simulink model "Assign_Task5and6"  (R2023a)
settings: Solver=ode1  StartTime=0.0  StopTime=30  FixedStep=Ts  MaxStep=Ts  RelTol=1e-3
model workspace (MAT data in the model file):
  wsw = 2000
values from neighbouring files (symbols this model uses):
  fg = 50    [Parameters.m]
  Rtpu = Xtpu/40    (= 0.00375)    [Parameters.m]
  S0non = 1000e6    (= 1000000000)    [Parameters.m]
  Svsc = 100e6    (= 100000000)    [Parameters.m]
  tonvsc = 1e-3    (= 0.001)    [Parameters.m]
  Ts = 20e-6    (= 2e-05)    [Parameters.m]
  Vhv = 22e3    (= 22000)    [Parameters.m]
  Vmv = 22e3    (= 22000)    [Parameters.m]
  wc1 = wsw1/10    (= 848.230016469)    [Parameters.m]
  wpq1 = wc1/10    (= 84.8230016469)    [Parameters.m]
  wsw1 = ksw1*2*pi*fg    (= 8482.30016469)    [Parameters.m]
  Xtpu = 0.15    [Parameters.m]
undefined symbols (not defined in the file or in its folder): D11, Delta, Kf, r, tfilt, theta0
libraries: simulink_extras x20, spsGroundLib x18, spsCurrentMeasurementLib x12, spsVoltageMeasurementLib x12, pid_lib x7, slpidlib x7, spsThreePhaseParallelRLCLoadLib x6, spsControlledVoltageSourceLib x6, powerlib_meascontrol x5, spsThreePhaseBreakerLib x4, eeTransforms x4, spsabctoAlphaBetaZeroLib x3
(part 1 of 3)
settings Model: Creator=Vinicius  LastModifiedBy=citcea
settings SolverCC: AlgebraicLoopSolver=TrustRegion
settings DataIOCC: InitialState=out_EMTsteady50VSC.xFinal  SaveOperatingPoint=on  SaveOutput=off  SignalLogging=off  DSMLogging=off  TimeSaveName=t
settings OptimizationCC: BlockReduction=off
settings ModelReferenceCC: EnableRefExpFcnMdlSchedulingChecks=on
settings RTWCC: BuildConfiguration=Faster Runs  DLArmComputeVersion=19.05

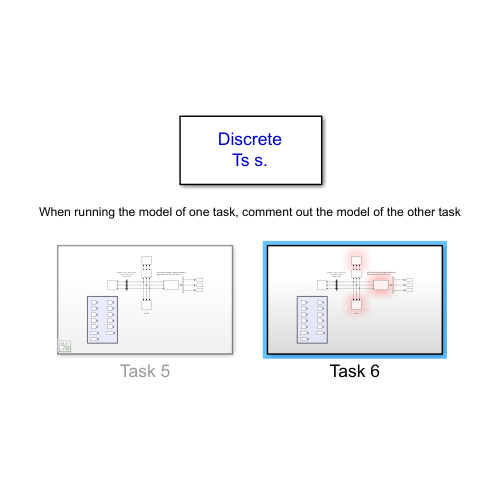
[thumbnail: Simulink's stored preview of the top-level diagram]
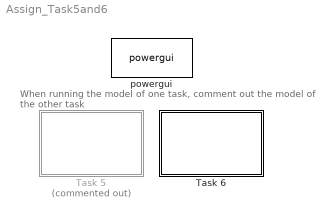
== system Assign_Task5and6 ==
  note: When running the model of one task, comment out the model of the other task
  Task 5 : Subsystem  Commented=on
  Task 6 : Subsystem
  powergui : spspowerguiLib/powergui  Priority=1  SimulationMode=Discrete  SampleTime=Ts  frequency=60  Iterations=50  frequencyindice=50  Pbase=100e6  ErrMax=0.0001  UnitsV=kV  UnitsW=MW  buscounter=0  FunctionMessages=off  echomessages=off  EnableUseOfTLC=off  CurrentSourceSwitches=off  DisableSnubberDevices=off  DisableRonSwitches=off  DisableVfSwitches=off  DisplayEquations=off  AutomaticDiscreteSolvers=off  SolverType=Tustin/Backward Euler (TBE)  Interpol=off  ExternalGateDelay=off  methode=off  Ts=100  x0status=blocks  SPID=on  SwTol=0  HookPort=off  NonlinearTolerance=1e-4  nMaxIteration=100  ContinueOnMaxIteration=off  RestoreLinks=warning  ResistiveCurrentMeasurement=off  Frange=[0:2:500]  Ylog=off  Xlog=on  ShowGrid=off  save=off  variable=ZData  structure=0  ZoomFFT=off  StartTime=0.0  cycles=1  DisplayStyle=1  fundamental=60  FreqAxis=off  MaxFrequency=1000  frequencyindicesteady=1  RmsSteady=1  display=off

== system Assign_Task5and6/Task 5 ==
  note: Variables
  note: Voltage, current, active power and reactive power measurement
  note: Load
  note: active and reactive power setpoints defined inside the VSC block
  Bus : Subsystem
  Bus Selector : BusSelector  OutputSignals=Pabc,Qabc,f
  Generator : Subsystem
      mask Display: disp('SG')
  Load bus 5 : spsThreePhaseParallelRLCLoadLib/Three-Phase Parallel RLC Load  LConnTagsString=A|B|C  Configuration=Y (grounded)  NominalVoltage=Vmv  Vabc=[1e3 1e3 1e3]  Vabcp=[1e3 1e3 1e3]  NominalFrequency=fg  UnbalancedPower=off  ActivePower=300e6  InductivePower=50e6  CapacitivePower=0  Pabc=[10e3 9e3 11e3]  QLabc=[100 90 110]  QCabc=[100 90 110]  Pabcp=[10e3 9e3 11e3]  QLabcp=[100 90 110]  QCabcp=[100 90 110]  Measurements=None  LoadType=constant PQ
  Three-Phase Parallel RLC Load2 : spsThreePhaseParallelRLCLoadLib/Three-Phase Parallel RLC Load  LConnTagsString=A|B|C  Configuration=Y (grounded)  NominalVoltage=Vmv  Vabc=[1 1 1]*Vhv  Vabcp=[1e3 1e3 1e3]  NominalFrequency=fg  UnbalancedPower=off  ActivePower=S0non*0.4  InductivePower=0  CapacitivePower=0  Pabc=[10 10 10]*1e6  QLabc=[1 1 1]*1e6  QCabc=[0 0 0]  Pabcp=[10e3 9e3 11e3]  QLabcp=[100 90 110]  QCabcp=[100 90 110]  Measurements=None  LoadType=constant Z
  Three-Phase Breaker1 : spsThreePhaseBreakerLib/Three-Phase Breaker  InitialState=open  SwitchA=on  SwitchB=on  SwitchC=on  SwitchTimes=4  External=off  BreakerResistance=0.001  SnubberResistance=1e7  SnubberCapacitance=inf  Measurements=None
  VSC : Subsystem  mask{fg=fg, Vhv=Vmv, Vmv=Vmv, Pconv=Svsc, Rtpu=Rtpu, Xtpu=Xtpu, wsw=wsw1, wn_pll=2*pi*80, wc=wc1, wpq=wpq1, koc=1.2}
      mask prompts: fg "AC grid frequency (Hz)"; Vhv "Grid-side voltage (V)(LL-rms)"; Vmv "Converter-side voltage (V)(LL-rms)"; Pconv "Converter nominal power (VA)"; Rtpu "Resistance seen by the converter (p.u)"; Xtpu "Reactance seen by the converter (p.u)"; wsw "Switching frequency (rad/s)"; wn_pll "PLL filter natural frequency"; wc "Current-control bandwidth (rad/s)"; wpq "PQ control bandwidth (rad/s)"; koc "Overcurrent factor (p.u)"
      mask init:
      | %% ----------------------VSC Parameters-------------------------- %%
      | Vmvpk = Vmv*sqrt(2)/sqrt(3);    % Converter-side voltage phase-to-ground peak-to-peak
      | Vhvpk = Vhv*sqrt(2)/sqrt(3);    % Grid-side voltage phase-to-ground peak-to-peak  
      | ksw = round(wsw/(2*pi*fg));      % Calculates switching ratio
      | Iconvbase = 2*Pconv/(3*Vmvpk);  % Converter base current (A)
      | Imax = koc*Iconvbase;   % Converter maximum output current
      | 
      | Xt = Xtpu*(Vmv^2/Pconv);        % p.u to (Ohms)
      | Lt = Xt/(2*pi*fg);              % p.u to (H)
      | Rt = Rtpu*(Vmv^2/Pconv);        % p.u. to (Ohms)
      | 
      | % ------------ PLL ------------- %
      | zeta_pll = 1/sqrt(2);           % Damping
      | kp_pll = 2*zeta_pll*wn_pll/(Vmvpk);
      | tau_pll = 2*zeta_pll/wn_pll;
      | 
      | % ------------ Inner-loop (current control) ------------ %
      | kp_c = Lt*wc; 
      | ti_c = Lt/Rt;
      | 
      | % -------- Outer-loop (voltage and/or power control)
      | % --- PQ closed-loop control ----
      | ti_pq = 1/wc;
      | kp_pq = 2/3*ti_pq*wpq*1/Vmvpk;
      | 
      | 
      | negseq_en = 0;
      mask DialogControl DescTextVar Prompt: Three-phase VSC model
      mask DialogControl Tab1 Prompt: Electrical parameters
      mask DialogControl Tab2 Prompt: Control parameters
      mask Display: disp('VSC')
  tag scope: Pvsc=global, Qvsc=global, fvsc=global
  wires:
  Bus Selector/1 -> [Pvsc]  "<Pabc>"
  Bus Selector/2 -> [Qvsc]  "<Qabc>"
  Bus Selector/3 -> [fvsc]  "<f>"
  VSC/1(m) -> Bus Selector/1
  connections:
  Load bus 5/LConn1 -- Three-Phase Breaker1/LConn1 -- VSC/LConn1 -- Bus/RConn1
  Load bus 5/LConn2 -- Bus/RConn2 -- VSC/LConn2 -- Three-Phase Breaker1/LConn2
  Generator/RConn1 -- Bus/LConn1
  Load bus 5/LConn3 -- Three-Phase Breaker1/LConn3 -- VSC/LConn3 -- Bus/RConn3
  Generator/RConn2 -- Bus/LConn2
  Generator/RConn3 -- Bus/LConn3
  Three-Phase Breaker1/RConn2 -- Three-Phase Parallel RLC Load2/LConn2
  Three-Phase Breaker1/RConn3 -- Three-Phase Parallel RLC Load2/LConn3
  Three-Phase Parallel RLC Load2/LConn1 -- Three-Phase Breaker1/RConn1

== system Assign_Task5and6/Task 6 ==
  note: Variables
  note: Voltage, current, active power and reactive power measurement
  note: Load
  note: active and reactive power setpoints defined inside the VSC block
  Bus : Subsystem
  Bus Selector : BusSelector  OutputSignals=Pabc,Qabc,f
  Generator : Subsystem
      mask Display: disp('SG')
  Load bus 5 : spsThreePhaseParallelRLCLoadLib/Three-Phase Parallel RLC Load  LConnTagsString=A|B|C  Configuration=Y (grounded)  NominalVoltage=Vmv  Vabc=[1e3 1e3 1e3]  Vabcp=[1e3 1e3 1e3]  NominalFrequency=fg  UnbalancedPower=off  ActivePower=300e6  InductivePower=50e6  CapacitivePower=0  Pabc=[10e3 9e3 11e3]  QLabc=[100 90 110]  QCabc=[100 90 110]  Pabcp=[10e3 9e3 11e3]  QLabcp=[100 90 110]  QCabcp=[100 90 110]  Measurements=None  LoadType=constant PQ
  Three-Phase Parallel RLC Load2 : spsThreePhaseParallelRLCLoadLib/Three-Phase Parallel RLC Load  LConnTagsString=A|B|C  Configuration=Y (grounded)  NominalVoltage=Vmv  Vabc=[1 1 1]*Vhv  Vabcp=[1e3 1e3 1e3]  NominalFrequency=fg  UnbalancedPower=off  ActivePower=S0non*0.4  InductivePower=0  CapacitivePower=0  Pabc=[10 10 10]*1e6  QLabc=[1 1 1]*1e6  QCabc=[0 0 0]  Pabcp=[10e3 9e3 11e3]  QLabcp=[100 90 110]  QCabcp=[100 90 110]  Measurements=None  LoadType=constant Z
  Three-Phase Breaker1 : spsThreePhaseBreakerLib/Three-Phase Breaker  InitialState=open  SwitchA=on  SwitchB=on  SwitchC=on  SwitchTimes=4  External=off  BreakerResistance=0.001  SnubberResistance=1e7  SnubberCapacitance=inf  Measurements=None
  VSC : Subsystem  mask{fg=fg, Vhv=Vmv, Vmv=Vmv, Pconv=Svsc, Rtpu=Rtpu, Xtpu=Xtpu, wsw=wsw1, wn_pll=2*pi*80, wc=wc1, wpq=wpq1, koc=1.2}
      mask prompts: fg "AC grid frequency (Hz)"; Vhv "Grid-side voltage (V)(LL-rms)"; Vmv "Converter-side voltage (V)(LL-rms)"; Pconv "Converter nominal power (VA)"; Rtpu "Resistance seen by the converter (p.u)"; Xtpu "Reactance seen by the converter (p.u)"; wsw "Switching frequency (rad/s)"; wn_pll "PLL filter natural frequency"; wc "Current-control bandwidth (rad/s)"; wpq "PQ control bandwidth (rad/s)"; koc "Overcurrent factor (p.u)"
      mask init: same as Assign_Task5and6/Task 5/VSC
      mask DialogControl DescTextVar Prompt: Three-phase VSC model
      mask DialogControl Tab1 Prompt: Electrical parameters
      mask DialogControl Tab2 Prompt: Control parameters
      mask Display: disp('VSC')
  tag scope: Pvsc=global, Qvsc=global, fvsc=global
  wires:
  Bus Selector/1 -> [Pvsc]  "<Pabc>"
  Bus Selector/2 -> [Qvsc]  "<Qabc>"
  Bus Selector/3 -> [fvsc]  "<f>"
  VSC/1(m) -> Bus Selector/1
  connections:
  Three-Phase Breaker1/LConn1 -- Bus/RConn1 -- Load bus 5/LConn1 -- VSC/LConn1
  Bus/RConn2 -- Three-Phase Breaker1/LConn2 -- Load bus 5/LConn2 -- VSC/LConn2
  Generator/RConn1 -- Bus/LConn1
  Three-Phase Breaker1/LConn3 -- Bus/RConn3 -- Load bus 5/LConn3 -- VSC/LConn3
  Generator/RConn2 -- Bus/LConn2
  Generator/RConn3 -- Bus/LConn3
  Three-Phase Breaker1/RConn2 -- Three-Phase Parallel RLC Load2/LConn2
  Three-Phase Breaker1/RConn3 -- Three-Phase Parallel RLC Load2/LConn3
  Three-Phase Parallel RLC Load2/LConn1 -- Three-Phase Breaker1/RConn1

== system Assign_Task5and6/Task 5/Bus ==
  Current Measurement : spsCurrentMeasurementLib/Current Measurement  PhasorSimulation=off  OutputType=Complex  PSBequivalent=0
  Current Measurement1 : spsCurrentMeasurementLib/Current Measurement  PhasorSimulation=off  OutputType=Complex  PSBequivalent=0
  Current Measurement2 : spsCurrentMeasurementLib/Current Measurement  PhasorSimulation=off  OutputType=Complex  PSBequivalent=0
  Ground3 : spsGroundLib/Ground  LConnTagsString=a
  Ground4 : spsGroundLib/Ground  LConnTagsString=a
  Ground5 : spsGroundLib/Ground  LConnTagsString=a
  Mux : Mux  Inputs=3
  Mux1 : Mux  Inputs=3
  Mux2 : Mux  Inputs=2
  "Power (3ph, Instantaneous)" : powerlib_meascontrol/Measurements/Power (3ph, Instantaneous)
  Voltage Measurement : spsVoltageMeasurementLib/Voltage Measurement  PhasorSimulation=off  OutputType=Complex  PSBequivalent=0
  Voltage Measurement2 : spsVoltageMeasurementLib/Voltage Measurement  PhasorSimulation=off  OutputType=Complex  PSBequivalent=0
  Voltage Measurement3 : spsVoltageMeasurementLib/Voltage Measurement  PhasorSimulation=off  OutputType=Complex  PSBequivalent=0
  A : PMIOPort  Side=Left
  B : PMIOPort  Port=2  Side=Left
  C : PMIOPort  Port=3  Side=Left
  a : PMIOPort  Port=4  Side=Right
  b : PMIOPort  Port=5  Side=Right
  c : PMIOPort  Port=6  Side=Right
  tag scope: Ig=global, PQ=global, Vg=global
  wires:
  Voltage Measurement3/1 -> Mux/3
  Voltage Measurement2/1 -> Mux/2
  Voltage Measurement/1 -> Mux/1
  Mux/1 -> [Vg], "Power (3ph, Instantaneous)"/1
  Current Measurement/1 -> Mux1/1
  Current Measurement1/1 -> Mux1/2
  Current Measurement2/1 -> Mux1/3
  Mux1/1 -> [Ig], "Power (3ph, Instantaneous)"/2
  "Power (3ph, Instantaneous)"/1 -> Mux2/1
  "Power (3ph, Instantaneous)"/2 -> Mux2/2
  Mux2/1 -> [PQ]
  connections:
  Ground5/LConn1 -- Voltage Measurement3/LConn2
  Current Measurement/RConn1 -- a/RConn1
  Voltage Measurement2/LConn1 -- Current Measurement1/LConn1 -- B/RConn1
  Voltage Measurement3/LConn1 -- Current Measurement2/LConn1 -- C/RConn1
  Voltage Measurement/LConn1 -- Current Measurement/LConn1 -- A/RConn1
  Ground3/LConn1 -- Voltage Measurement/LConn2
  Ground4/LConn1 -- Voltage Measurement2/LConn2
  Current Measurement1/RConn1 -- b/RConn1
  Current Measurement2/RConn1 -- c/RConn1

== system Assign_Task5and6/Task 5/Generator ==
  note: The Snubber should be at least equal to 1% of the machine power to avoid numerical oscillations
  note: Nomenclature:
      |
      | Pm = mechanical power provided to the generator
      | Tm = mechanical torque provided to the generator
      | wm = mechanical speed in p.u
      | dw = speed variation (wm-1) in p.u
      | Efd = Exciter output voltage (generator field voltage)
      | Ifd = Exciter output current (generator field current)
      | Vt = Generator terminal voltage
      | It = Generator terminal current
      | Vref = Voltage regulator reference signal
  note: Synchronous Machine Model according to ENTSO-E
  note: The mechanical power should be changed here in this constant and also in the turbine parameters
  Abs1 : Abs  SaturateOnIntegerOverflow=off
  Abs2 : Abs  SaturateOnIntegerOverflow=off
  Bus Selector : BusSelector  OutputSignals=dw,w,vq,vd,iq,id,Peo,Te,ifd
  Divide : Product  Inputs=*/
  Exciter : Subsystem  mask{K=200, Ta=3, Tb=10, Te=0.05, Emin=-4, Emax=4, Vf0=1.30534}
      mask prompts: K "Controller gain (K)"; Ta "Filter derivative time constant (Ta)(sec)"; Tb "Filter delay time (Tb)(sec)"; Te "Exciter time constant (Te)(sec)"; Emin "Controller minimum output (Emin)"; Emax "Controller maximum output (Emax)"; Vf0 "Initial output (p.u)"
      mask Display:
      | disp('AVR')
      | 
      | port_label('input',1,'Vref')
      | port_label('input',2,'Vc')
      | 
      | port_label('output',1,'Efd')
  Mech power (p.u) : Constant  Value=0.350  VectorParams1D=off
  Real-Imag to Complex : RealImagToComplex
  Real-Imag to Complex1 : RealImagToComplex
  Scope : Scope
  Snubber : spsThreePhaseParallelRLCLoadLib/Three-Phase Parallel RLC Load  LConnTagsString=A|B|C  Configuration=Y (grounded)  NominalVoltage=Vmv  Vabc=[1 1 1]*Vmv  Vabcp=[1e3 1e3 1e3]  NominalFrequency=fg  UnbalancedPower=off  ActivePower=0.05*S0non  InductivePower=0  CapacitivePower=0  Pabc=[10e3 10e3 10e3]  QLabc=[0 0 0]  QCabc=[0 0 0]  Pabcp=[10e3 9e3 11e3]  QLabcp=[100 90 110]  QCabcp=[100 90 110]  Measurements=None  LoadType=constant Z
  Synchronous machine : spsSynchronousMachinepuStandardLib/Synchronous Machine pu Standard  PresetModel=No  MechanicalLoad=Mechanical power Pm  ShowDetailedParameters=on  RotorType=Salient-pole  Units=per unit standard parameters  MeasurementBus=on  NominalParameters=[S0non Vmv fg]  Reactances1=[ 1.81, 0.3, 0.23, 1.76, 0.65, 0.25, 0.15 ]  Reactances2=[2.0 0.35 0.25 1.8 0.3 0.15]  dAxisTimeConstants=Short-circuit  qAxisTimeConstants=Short-circuit  TimeConstants1="[ 4.4849  0.0681  0.1  ]"  TimeConstants2=[ 8.0, 0.03, 1.0, 0.07 ]  TimeConstants3="[  4.49  0.0681  0.0513  ]"  TimeConstants4=[ 8.0, 0.03, 0.3371, 0.0295 ]  TimeConstants5=[ 1.01, 0.053, 0.1 ]  TimeConstants6=[ 1.3201, 0.023, 1.0, 0.07 ]  TimeConstants7=[0.9 0.03 0.05]  TimeConstants8=[ 1.3201, 0.0231, 0.3371, 0.0295 ]  StatorResistance=0.01  Mechanical=[6 0 2]  PolePairs=20  InitialConditions=[0 -60.0721 0.353553 0.353553 0.353553 -8.1301 -128.13 111.87 1.30534]  SetSaturation=off  Saturation=[0.6404,0.7127,0.8441,0.9214,0.9956,1.082,1.19,1.316,1.457;0.7,0.7698,0.8872,0.9466,0.9969,1.046,1.1,1.151,1.201]  LoadFlowParameters=[2 47500000 0 0 0]  TsPowergui=0  TsBlock=-1  IterativeModel=Trapezoidal non iterative  IterativeDiscreteModel=Trapezoidal non iterative  BusType=swing  Pref=475e6  Qref=0  Qmin=-inf  Qmax=inf  PLF=0  QLF=0
  Turbine without governor : Subsystem  mask{R=0.05, T1=0.5, T2=3, T3=10, Dt=0, Vmin=0, Vmax=10, P0=0.351}
      mask prompts: R "Controller droop (R)"; T1 "Governor time constant (T1)(sec)"; T2 "Turbine derivative time constant (T2)(sec)"; T3 "Turbine delay time constant (T3)(sec)"; Dt "Frictional losses factor (Dt)"; Vmin "Minimum gate limit (Vmin)(p.u)"; Vmax "Maximum gate limit (Vmax)(p.u)"; P0 "Initial power (p.u)"
      mask Display:
      | disp('Turbine')
      | 
      | port_label('input',1,'Pref')
      | 
      | port_label('output',1,'Pm')
  Voltage ref (p.u) : Constant  Value=1.0
  A : PMIOPort  Side=Right
  B : PMIOPort  Port=2  Side=Right
  C : PMIOPort  Port=3  Side=Right
  tag scope: Efd=global, Ifd=global, It=global, Pe=global, Pm=global, Te=global, Tm=global, Vt=global, dw=global, wm=global
  wires:
  Exciter/1(Efd) -> Synchronous machine/2, [Efd]
  Voltage ref (p.u)/1 -> Exciter/1(Vref)
  Turbine without governor/1(Pm) -> Synchronous machine/1, [Pm]
  Mech power (p.u)/1 -> Turbine without governor/1(RefL)
  [Pm] -> Divide/1
  [wm] -> Divide/2
  Divide/1 -> [Tm]
  Bus Selector/4 -> Real-Imag to Complex/2  "<vd>"
  Abs2/1 -> [It]
  Real-Imag to Complex1/1 -> Abs2/1
  Real-Imag to Complex/1 -> Abs1/1
  Bus Selector/6 -> Real-Imag to Complex1/2  "<id>"
  Bus Selector/2 -> Scope/1, [wm]  "<w>"
  Bus Selector/8 -> [Te]  "<Te>"
  Bus Selector/3 -> Real-Imag to Complex/1  "<vq>"
  Bus Selector/7 -> [Pe]  "<Peo>"
  Bus Selector/5 -> Real-Imag to Complex1/1  "<iq>"
  Synchronous machine/1 -> Bus Selector/1
  Bus Selector/9 -> [Ifd]  "<ifd>"
  Abs1/1 -> [Vt]
  [Vt] -> Exciter/2(Vt)
  Bus Selector/1 -> [dw]  "<dw>"
  connections:
  B/RConn1 -- Synchronous machine/RConn2 -- Snubber/LConn2
  C/RConn1 -- Synchronous machine/RConn3 -- Snubber/LConn3
  Snubber/LConn1 -- Synchronous machine/RConn1 -- A/RConn1

== system Assign_Task5and6/Task 5/VSC ==
  note: Load convention used:
      | positive power = converter absorbs power from the grid
      | negative power = converter injects power into the grid
  Block : Step  Time=4*tonvsc  Before=1  After=0  SampleTime=0
  Electrical part : Subsystem  VariantControl=EMT_AVG
      settings: PortSchema="{\"entries\":[{\"content\":{\"sides\":[{\"content\":{\"connectorIds\":[\"LConn1\",\"LConn2\",\"LConn3\"]},\"type\":\"ConnectorPlacement.EquallySpacedRectSide\",\"uuid\":\"96043b84-a665-4cb2-a938-d6633d7ee474\"},{\"content\":{\"connectorIds\":[\"In1\"],\"side\":\"RIGHT\"},\"type\":\"ConnectorPlacement.EquallySpacedRectSide\",\"uuid\":\"064d463f-c23a-42ac-89ce-8dea3d446214\"},{\"content\":{\"connectorIds\":[],\"side\":\"TOP\"},\"type\":\"ConnectorPlacement.EquallySpacedRectSide\",\"uuid\":\"95ef669c-c6ed-44c3-8b69-447906728b6d\"}]},\"type\":\"ConnectorPlacement.EquallySpacedConnector\",\"uuid\":\"ea66db09-64d7-4d7e-ba7b-d769c56e2dbd\"}],\"packageUris\":[\"http://schema.mathworks.com/mf0/Connector/19700101\"],\"version\":\"1.0\"}"
  NOT : Logic  Operator=NOT  IconShape=distinctive  AllPortsSameDT=off  OutDataTypeStr=boolean
  Pset : Step  Time=4*tonvsc  After=-Svsc*0.2  SampleTime=0
  Qset : Step  Time=tonvsc  After=0  SampleTime=0
  Three-Phase Breaker : spsThreePhaseBreakerLib/Three-Phase Breaker  InitialState=open  SwitchA=on  SwitchB=on  SwitchC=on  SwitchTimes="[1/60  5/60]"  External=on  BreakerResistance=0.001  SnubberResistance=1e7  SnubberCapacitance=inf  Measurements=None
  VI measurement : Subsystem
      settings: PortSchema="{\"entries\":[{\"content\":{\"sides\":[{\"content\":{\"connectorIds\":[\"LConn1\",\"LConn2\",\"LConn3\"]},\"type\":\"ConnectorPlacement.EquallySpacedRectSide\",\"uuid\":\"d0d5b0b8-afec-4f90-9eba-536a06b10059\"},{\"content\":{\"connectorIds\":[\"RConn1\",\"RConn2\",\"RConn3\"],\"side\":\"RIGHT\"},\"type\":\"ConnectorPlacement.EquallySpacedRectSide\",\"uuid\":\"adc1b68d-6172-4507-b54b-9373921355a1\"},{\"content\":{\"connectorIds\":[\"Out1\",\"Out2\"],\"side\":\"TOP\"},\"type\":\"ConnectorPlacement.EquallySpacedRectSide\",\"uuid\":\"8c5adf07-e95b-4907-94c3-1b2a47d47f40\"}]},\"type\":\"ConnectorPlacement.EquallySpacedConnector\",\"uuid\":\"87d0b20f-8f85-4790-a611-3415e642a83a\"}],\"packageUris\":[\"http://schema.mathworks.com/mf0/Connector/R2020b\"],\"version\":\"1.0\"}"
  VSC Control : Subsystem
      settings: PortSchema="{\"entries\":[{\"content\":{\"sides\":[{\"content\":{\"connectorIds\":[\"In1\",\"In2\",\"In3\",\"In4\",\"In5\"]},\"type\":\"ConnectorPlacement.EquallySpacedRectSide\",\"uuid\":\"cada8d9e-53e0-4197-9386-6c7b6ea13844\"},{\"content\":{\"connectorIds\":[\"Out1\"],\"side\":\"RIGHT\"},\"type\":\"ConnectorPlacement.EquallySpacedRectSide\",\"uuid\":\"f237b52a-0d77-45c0-937d-32cafba1283e\"},{\"content\":{\"connectorIds\":[\"Out2\"],\"side\":\"TOP\"},\"type\":\"ConnectorPlacement.EquallySpacedRectSide\",\"uuid\":\"e6f268b5-5f09-49a6-9529-b1aeebd5f021\"}]},\"type\":\"ConnectorPlacement.EquallySpacedConnector\",\"uuid\":\"4d1d2957-2eb9-4111-8c87-957e800b2b0b\"}],\"packageUris\":[\"http://schema.mathworks.com/mf0/Connector/19700101\"],\"version\":\"1.0\"}"
  output signals : Subsystem
  A : PMIOPort  Side=Left
  B : PMIOPort  Port=2  Side=Left
  C : PMIOPort  Port=3  Side=Left
  m : Outport
  wires:
  NOT/1 -> Three-Phase Breaker/1
  VSC Control/1(Ref) -> Electrical part/1(Ref)
  [Is] -> VSC Control/3(Iabc)
  [Vs] -> VSC Control/2(Vabc)
  Block/1 -> VSC Control/1(Block), NOT/1
  [Vs] -> output signals/1(Vs)
  [Is] -> output signals/2(Is)
  VSC Control/2(m) -> output signals/3(control)
  output signals/1(m) -> m/1
  VI measurement/1(Vs) -> [Vs]
  VI measurement/2(Is) -> [Is]
  Pset/1 -> VSC Control/4(Pset)
  Qset/1 -> VSC Control/5(Qset)
  connections:
  Electrical part/LConn3 -- Three-Phase Breaker/LConn3
  Electrical part/LConn2 -- Three-Phase Breaker/LConn2
  Electrical part/LConn1 -- Three-Phase Breaker/LConn1
  Three-Phase Breaker/RConn1 -- VI measurement/RConn1
  Three-Phase Breaker/RConn2 -- VI measurement/RConn2
  Three-Phase Breaker/RConn3 -- VI measurement/RConn3
  VI measurement/LConn3 -- C/RConn1
  A/RConn1 -- VI measurement/LConn1
  B/RConn1 -- VI measurement/LConn2

== system Assign_Task5and6/Task 6/Bus ==
  Current Measurement : spsCurrentMeasurementLib/Current Measurement  PhasorSimulation=off  OutputType=Complex  PSBequivalent=0
  Current Measurement1 : spsCurrentMeasurementLib/Current Measurement  PhasorSimulation=off  OutputType=Complex  PSBequivalent=0
  Current Measurement2 : spsCurrentMeasurementLib/Current Measurement  PhasorSimulation=off  OutputType=Complex  PSBequivalent=0
  Ground3 : spsGroundLib/Ground  LConnTagsString=a
  Ground4 : spsGroundLib/Ground  LConnTagsString=a
  Ground5 : spsGroundLib/Ground  LConnTagsString=a
  Mux : Mux  Inputs=3
  Mux1 : Mux  Inputs=3
  Mux2 : Mux  Inputs=2
  "Power (3ph, Instantaneous)" : spsPower3phInstantaneousLib/Power (3ph, Instantaneous)
  Voltage Measurement : spsVoltageMeasurementLib/Voltage Measurement  PhasorSimulation=off  OutputType=Complex  PSBequivalent=0
  Voltage Measurement2 : spsVoltageMeasurementLib/Voltage Measurement  PhasorSimulation=off  OutputType=Complex  PSBequivalent=0
  Voltage Measurement3 : spsVoltageMeasurementLib/Voltage Measurement  PhasorSimulation=off  OutputType=Complex  PSBequivalent=0
  A : PMIOPort  Side=Left
  B : PMIOPort  Port=2  Side=Left
  C : PMIOPort  Port=3  Side=Left
  a : PMIOPort  Port=4  Side=Right
  b : PMIOPort  Port=5  Side=Right
  c : PMIOPort  Port=6  Side=Right
  tag scope: Ig=global, PQ=global, Vg=global
  wires:
  Voltage Measurement3/1 -> Mux/3
  Voltage Measurement2/1 -> Mux/2
  Voltage Measurement/1 -> Mux/1
  Mux/1 -> [Vg], "Power (3ph, Instantaneous)"/1
  Current Measurement/1 -> Mux1/1
  Current Measurement1/1 -> Mux1/2
  Current Measurement2/1 -> Mux1/3
  Mux1/1 -> [Ig], "Power (3ph, Instantaneous)"/2
  "Power (3ph, Instantaneous)"/1 -> Mux2/1
  "Power (3ph, Instantaneous)"/2 -> Mux2/2
  Mux2/1 -> [PQ]
  connections:
  Ground5/LConn1 -- Voltage Measurement3/LConn2
  Current Measurement/RConn1 -- a/RConn1
  Voltage Measurement2/LConn1 -- Current Measurement1/LConn1 -- B/RConn1
  Voltage Measurement3/LConn1 -- Current Measurement2/LConn1 -- C/RConn1
  Voltage Measurement/LConn1 -- Current Measurement/LConn1 -- A/RConn1
  Ground3/LConn1 -- Voltage Measurement/LConn2
  Ground4/LConn1 -- Voltage Measurement2/LConn2
  Current Measurement1/RConn1 -- b/RConn1
  Current Measurement2/RConn1 -- c/RConn1

== system Assign_Task5and6/Task 6/Generator ==
  note: The Snubber should be at least equal to 1% of the machine power to avoid numerical oscillations
  note: Nomenclature:
      |
      | Pm = mechanical power provided to the generator
      | Tm = mechanical torque provided to the generator
      | wm = mechanical speed in p.u
      | dw = speed variation (wm-1) in p.u
      | Efd = Exciter output voltage (generator field voltage)
      | Ifd = Exciter output current (generator field current)
      | Vt = Generator terminal voltage
      | It = Generator terminal current
      | Vref = Voltage regulator reference signal
  note: Synchronous Machine Model according to ENTSO-E
  note: The mechanical power should be changed here in this constant and also in the turbine parameters
  Abs1 : Abs  SaturateOnIntegerOverflow=off
  Abs2 : Abs  SaturateOnIntegerOverflow=off
  Bus Selector : BusSelector  OutputSignals=dw,w,vq,vd,iq,id,Peo,Te,ifd
  Divide : Product  Inputs=*/
  Exciter : Subsystem  mask{K=200, Ta=3, Tb=10, Te=0.05, Emin=-4, Emax=4, Vf0=1.30534}
      mask prompts: K "Controller gain (K)"; Ta "Filter derivative time constant (Ta)(sec)"; Tb "Filter delay time (Tb)(sec)"; Te "Exciter time constant (Te)(sec)"; Emin "Controller minimum output (Emin)"; Emax "Controller maximum output (Emax)"; Vf0 "Initial output (p.u)"
      mask Display:
      | disp('AVR')
      | 
      | port_label('input',1,'Vref')
      | port_label('input',2,'Vc')
      | 
      | port_label('output',1,'Efd')
  Mech power (p.u) : Constant  Value=0.350  VectorParams1D=off
  Real-Imag to Complex : RealImagToComplex
  Real-Imag to Complex1 : RealImagToComplex
  Scope : Scope
  Snubber : spsThreePhaseParallelRLCLoadLib/Three-Phase Parallel RLC Load  LConnTagsString=A|B|C  Configuration=Y (grounded)  NominalVoltage=Vmv  Vabc=[1 1 1]*Vmv  Vabcp=[1e3 1e3 1e3]  NominalFrequency=fg  UnbalancedPower=off  ActivePower=0.05*S0non  InductivePower=0  CapacitivePower=0  Pabc=[10e3 10e3 10e3]  QLabc=[0 0 0]  QCabc=[0 0 0]  Pabcp=[10e3 9e3 11e3]  QLabcp=[100 90 110]  QCabcp=[100 90 110]  Measurements=None  LoadType=constant Z
  Synchronous machine : spsSynchronousMachinepuStandardLib/Synchronous Machine pu Standard  PresetModel=No  MechanicalLoad=Mechanical power Pm  ShowDetailedParameters=on  RotorType=Salient-pole  Units=per unit standard parameters  MeasurementBus=on  NominalParameters=[S0non Vmv fg]  Reactances1=[ 1.81, 0.3, 0.23, 1.76, 0.65, 0.25, 0.15 ]  Reactances2=[2.0 0.35 0.25 1.8 0.3 0.15]  dAxisTimeConstants=Short-circuit  qAxisTimeConstants=Short-circuit  TimeConstants1="[ 4.4849  0.0681  0.1  ]"  TimeConstants2=[ 8.0, 0.03, 1.0, 0.07 ]  TimeConstants3="[  4.49  0.0681  0.0513  ]"  TimeConstants4=[ 8.0, 0.03, 0.3371, 0.0295 ]  TimeConstants5=[ 1.01, 0.053, 0.1 ]  TimeConstants6=[ 1.3201, 0.023, 1.0, 0.07 ]  TimeConstants7=[0.9 0.03 0.05]  TimeConstants8=[ 1.3201, 0.0231, 0.3371, 0.0295 ]  StatorResistance=0.01  Mechanical=[6 0 2]  PolePairs=20  InitialConditions=[0 -60.0721 0.353553 0.353553 0.353553 -8.1301 -128.13 111.87 1.30534]  SetSaturation=off  Saturation=[0.6404,0.7127,0.8441,0.9214,0.9956,1.082,1.19,1.316,1.457;0.7,0.7698,0.8872,0.9466,0.9969,1.046,1.1,1.151,1.201]  LoadFlowParameters=[2 47500000 0 0 0]  TsPowergui=0  TsBlock=-1  IterativeModel=Trapezoidal non iterative  IterativeDiscreteModel=Trapezoidal non iterative  BusType=swing  Pref=475e6  Qref=0  Qmin=-inf  Qmax=inf  PLF=0  QLF=0
  Turbine without governor : Subsystem  mask{R=0.05, T1=0.5, T2=3, T3=10, Dt=0, Vmin=0, Vmax=10, P0=0.351}
      mask prompts: R "Controller droop (R)"; T1 "Governor time constant (T1)(sec)"; T2 "Turbine derivative time constant (T2)(sec)"; T3 "Turbine delay time constant (T3)(sec)"; Dt "Frictional losses factor (Dt)"; Vmin "Minimum gate limit (Vmin)(p.u)"; Vmax "Maximum gate limit (Vmax)(p.u)"; P0 "Initial power (p.u)"
      mask Display:
      | disp('Turbine')
      | 
      | port_label('input',1,'Pref')
      | 
      | port_label('output',1,'Pm')
  Voltage ref (p.u) : Constant  Value=1.0
  A : PMIOPort  Side=Right
  B : PMIOPort  Port=2  Side=Right
  C : PMIOPort  Port=3  Side=Right
  tag scope: Efd=global, Ifd=global, It=global, Pe=global, Pm=global, Te=global, Tm=global, Vt=global, dw=global, wm=global
  wires:
  Exciter/1(Efd) -> Synchronous machine/2, [Efd]
  Voltage ref (p.u)/1 -> Exciter/1(Vref)
  Turbine without governor/1(Pm) -> Synchronous machine/1, [Pm]
  Mech power (p.u)/1 -> Turbine without governor/1(RefL)
  [Pm] -> Divide/1
  [wm] -> Divide/2
  Divide/1 -> [Tm]
  Bus Selector/4 -> Real-Imag to Complex/2  "<vd>"
  Abs2/1 -> [It]
  Real-Imag to Complex1/1 -> Abs2/1
  Real-Imag to Complex/1 -> Abs1/1
  Bus Selector/6 -> Real-Imag to Complex1/2  "<id>"
  Bus Selector/2 -> Scope/1, [wm]  "<w>"
  Bus Selector/8 -> [Te]  "<Te>"
  Bus Selector/3 -> Real-Imag to Complex/1  "<vq>"
  Bus Selector/7 -> [Pe]  "<Peo>"
  Bus Selector/5 -> Real-Imag to Complex1/1  "<iq>"
  Synchronous machine/1 -> Bus Selector/1
  Bus Selector/9 -> [Ifd]  "<ifd>"
  Abs1/1 -> [Vt]
  [Vt] -> Exciter/2(Vt)
  Bus Selector/1 -> [dw]  "<dw>"
  connections:
  B/RConn1 -- Synchronous machine/RConn2 -- Snubber/LConn2
  C/RConn1 -- Synchronous machine/RConn3 -- Snubber/LConn3
  Snubber/LConn1 -- Synchronous machine/RConn1 -- A/RConn1

== system Assign_Task5and6/Task 6/VSC ==
  note: droop signal goes here
  note: Load convention used:
      | positive power = converter absorbs power from the grid
      | negative power = converter injects power into the grid
  Block : Step  Time=4*tonvsc  Before=1  After=0  SampleTime=0
  Electrical part : Subsystem  VariantControl=EMT_AVG
      settings: PortSchema="{\"entries\":[{\"content\":{\"sides\":[{\"content\":{\"connectorIds\":[\"LConn1\",\"LConn2\",\"LConn3\"]},\"type\":\"ConnectorPlacement.EquallySpacedRectSide\",\"uuid\":\"96043b84-a665-4cb2-a938-d6633d7ee474\"},{\"content\":{\"connectorIds\":[\"In1\"],\"side\":\"RIGHT\"},\"type\":\"ConnectorPlacement.EquallySpacedRectSide\",\"uuid\":\"064d463f-c23a-42ac-89ce-8dea3d446214\"},{\"content\":{\"connectorIds\":[],\"side\":\"TOP\"},\"type\":\"ConnectorPlacement.EquallySpacedRectSide\",\"uuid\":\"95ef669c-c6ed-44c3-8b69-447906728b6d\"}]},\"type\":\"ConnectorPlacement.EquallySpacedConnector\",\"uuid\":\"ea66db09-64d7-4d7e-ba7b-d769c56e2dbd\"}],\"packageUris\":[\"http://schema.mathworks.com/mf0/Connector/19700101\"],\"version\":\"1.0\"}"
  NOT : Logic  Operator=NOT  IconShape=distinctive  AllPortsSameDT=off  OutDataTypeStr=boolean
  Pset : Step  Time=4*tonvsc  After=-Svsc*0.2  SampleTime=0
  Qset : Step  Time=tonvsc  After=0  SampleTime=0
  Three-Phase Breaker : spsThreePhaseBreakerLib/Three-Phase Breaker  InitialState=open  SwitchA=on  SwitchB=on  SwitchC=on  SwitchTimes="[1/60  5/60]"  External=on  BreakerResistance=0.001  SnubberResistance=1e7  SnubberCapacitance=inf  Measurements=None
  VI measurement : Subsystem
      settings: PortSchema="{\"entries\":[{\"content\":{\"sides\":[{\"content\":{\"connectorIds\":[\"LConn1\",\"LConn2\",\"LConn3\"]},\"type\":\"ConnectorPlacement.EquallySpacedRectSide\",\"uuid\":\"d0d5b0b8-afec-4f90-9eba-536a06b10059\"},{\"content\":{\"connectorIds\":[\"RConn1\",\"RConn2\",\"RConn3\"],\"side\":\"RIGHT\"},\"type\":\"ConnectorPlacement.EquallySpacedRectSide\",\"uuid\":\"adc1b68d-6172-4507-b54b-9373921355a1\"},{\"content\":{\"connectorIds\":[\"Out1\",\"Out2\"],\"side\":\"TOP\"},\"type\":\"ConnectorPlacement.EquallySpacedRectSide\",\"uuid\":\"8c5adf07-e95b-4907-94c3-1b2a47d47f40\"}]},\"type\":\"ConnectorPlacement.EquallySpacedConnector\",\"uuid\":\"87d0b20f-8f85-4790-a611-3415e642a83a\"}],\"packageUris\":[\"http://schema.mathworks.com/mf0/Connector/R2020b\"],\"version\":\"1.0\"}"
  VSC Control : Subsystem
      settings: PortSchema="{\"entries\":[{\"content\":{\"sides\":[{\"content\":{\"connectorIds\":[\"In1\",\"In2\",\"In3\",\"In4\",\"In5\"]},\"type\":\"ConnectorPlacement.EquallySpacedRectSide\",\"uuid\":\"cada8d9e-53e0-4197-9386-6c7b6ea13844\"},{\"content\":{\"connectorIds\":[\"Out1\"],\"side\":\"RIGHT\"},\"type\":\"ConnectorPlacement.EquallySpacedRectSide\",\"uuid\":\"f237b52a-0d77-45c0-937d-32cafba1283e\"},{\"content\":{\"connectorIds\":[\"Out2\"],\"side\":\"TOP\"},\"type\":\"ConnectorPlacement.EquallySpacedRectSide\",\"uuid\":\"e6f268b5-5f09-49a6-9529-b1aeebd5f021\"}]},\"type\":\"ConnectorPlacement.EquallySpacedConnector\",\"uuid\":\"4d1d2957-2eb9-4111-8c87-957e800b2b0b\"}],\"packageUris\":[\"http://schema.mathworks.com/mf0/Connector/19700101\"],\"version\":\"1.0\"}"
  output signals : Subsystem
  A : PMIOPort  Side=Left
  B : PMIOPort  Port=2  Side=Left
  C : PMIOPort  Port=3  Side=Left
  m : Outport
  wires:
  NOT/1 -> Three-Phase Breaker/1
  VSC Control/1(Ref) -> Electrical part/1(Ref)
  [Is] -> VSC Control/3(Iabc)
  [Vs] -> VSC Control/2(Vabc)
  Block/1 -> VSC Control/1(Block), NOT/1
  [Vs] -> output signals/1(Vs)
  [Is] -> output signals/2(Is)
  VSC Control/2(m) -> output signals/3(control)
  output signals/1(m) -> m/1
  VI measurement/1(Vs) -> [Vs]
  VI measurement/2(Is) -> [Is]
  Pset/1 -> VSC Control/4(Pset)
  Qset/1 -> VSC Control/5(Qset)
  connections:
  Electrical part/LConn3 -- Three-Phase Breaker/LConn3
  Electrical part/LConn2 -- Three-Phase Breaker/LConn2
  Electrical part/LConn1 -- Three-Phase Breaker/LConn1
  Three-Phase Breaker/RConn1 -- VI measurement/RConn1
  Three-Phase Breaker/RConn2 -- VI measurement/RConn2
  Three-Phase Breaker/RConn3 -- VI measurement/RConn3
  VI measurement/LConn3 -- C/RConn1
  A/RConn1 -- VI measurement/LConn1
  B/RConn1 -- VI measurement/LConn2

== system Assign_Task5and6/Task 5/Generator/Exciter ==
  note: The controller parameters provided by ENTSO-E
      | define different names for the parameters:
      |
      | ENTSO-E = IEEE Std 421.5-2005
      | Ta = Tc
      | Tb = Tb
      | K = Ka
      | Te = Ta
      | Emax = Vrmax
      | Emin = Vrmin
  note: The exciter model provided by ENTSO-E most similar to the IEEE is the Type AC4A excitation system model
  Vref : Inport
  Vt : Inport  Port=2
  Constant : Constant  Value=Vf0/K
  Saturation : Saturate  UpperLimit=Emax  LowerLimit=Emin
  Sum : Sum  Inputs=++-
  Transfer Fcn (with initial outputs) : simulink_extras/Additional Linear/Transfer Fcn (with initial outputs)  N=[K]  D=[Te 1]  Y0=Vf0  U0=Vf0/K
  Transfer Fcn (with initial outputs)1 : simulink_extras/Additional Linear/Transfer Fcn (with initial outputs)  N=[Ta 1]  D=[Tb 1]  Y0=Vf0/K  U0=Vf0/K
  Efd : Outport
  wires:
  Saturation/1 -> Efd/1
  Transfer Fcn (with initial outputs)1/1 -> Transfer Fcn (with initial outputs)/1
  Sum/1 -> Transfer Fcn (with initial outputs)1/1
  Transfer Fcn (with initial outputs)/1 -> Saturation/1
  Vt/1 -> Sum/3
  Vref/1 -> Sum/2
  Constant/1 -> Sum/1

== system Assign_Task5and6/Task 5/Generator/Turbine without governor ==
  note: mechanical power
  RefL : Inport
  Saturation : Saturate  UpperLimit=Vmax  LowerLimit=Vmin
  Saturation1 : Saturate  UpperLimit=1
  Transfer Fcn (with initial outputs)1 : simulink_extras/Additional Linear/Transfer Fcn (with initial outputs)  N=[T2 1]  D=[T3 1]  Y0=P0  U0=P0
  Transfer Fcn (with initial outputs)2 : simulink_extras/Additional Linear/Transfer Fcn (with initial outputs)  N=[1]  D=[T1 1]  Y0=P0  U0=P0
  Pm : Outport
  wires:
  Transfer Fcn (with initial outputs)1/1 -> Saturation1/1
  Saturation/1 -> Transfer Fcn (with initial outputs)1/1
  Transfer Fcn (with initial outputs)2/1 -> Saturation/1
  RefL/1 -> Transfer Fcn (with initial outputs)2/1
  Saturation1/1 -> Pm/1

== system Assign_Task5and6/Task 5/VSC/Electrical part ==
  Ref : Inport
  Controlled Voltage Source3 : spsControlledVoltageSourceLib/Controlled Voltage Source  Initialize=off  Source_Type=AC  Amplitude=Vhvpk  Phase=0  Frequency=fg  Measurements=None
  Controlled Voltage Source4 : spsControlledVoltageSourceLib/Controlled Voltage Source  Initialize=off  Source_Type=AC  Amplitude=Vhvpk  Phase=-2*pi/3  Frequency=fg  Measurements=None
  Controlled Voltage Source5 : spsControlledVoltageSourceLib/Controlled Voltage Source  Initialize=off  Source_Type=AC  Amplitude=Vhvpk  Phase=-4*pi/3  Frequency=fg  Measurements=None
  Demux1 : Demux  Outputs=3
  Ground : spsGroundLib/Ground  LConnTagsString=a
  Ground4 : spsGroundLib/Ground  LConnTagsString=a
  Ground5 : spsGroundLib/Ground  LConnTagsString=a
  Three-Phase Transformer (Two Windings) : spsThreePhaseTransformerTwoWindingsLib/Three-Phase Transformer (Two Windings)  Winding1Connection=Yg  Winding2Connection=Delta (D11)  CoreType=Three single-phase transformers  SetSaturation=off  Hysteresis=off  DataFile='hysteresis'  SetInitialFlux=off  Measurements=None  UNITS=pu  NominalPower=[Pconv , fg ]  Winding1=[Vhv, Rtpu/2, Xtpu/2]  Winding2=[Vmv, Rtpu/2, Xtpu/2]  Rm=5000  Lm=5000  L0=0.5  Saturation=[ 0,0 ; 0.0024,1.2 ; 1.0,1.52 ]  InitialFluxes=[ 0.8 , -0.8 , 0.7 ]  BreakLoop=off  DiscreteSolver=Trapezoidal iterative  DataType=off  TransfoNumber=1
  A : PMIOPort  Side=Left
  B : PMIOPort  Port=2  Side=Left
  C : PMIOPort  Port=3  Side=Left
  wires:
  Ref/1 -> Demux1/1
  Demux1/1 -> Controlled Voltage Source3/1
  Demux1/2 -> Controlled Voltage Source4/1
  Demux1/3 -> Controlled Voltage Source5/1
  connections:
  Ground/LConn1 -- Controlled Voltage Source3/LConn1
  Ground4/LConn1 -- Controlled Voltage Source4/LConn1
  Ground5/LConn1 -- Controlled Voltage Source5/LConn1
  Three-Phase Transformer (Two Windings)/LConn1 -- A/RConn1
  B/RConn1 -- Three-Phase Transformer (Two Windings)/LConn2
  Three-Phase Transformer (Two Windings)/LConn3 -- C/RConn1
  Three-Phase Transformer (Two Windings)/RConn1 -- Controlled Voltage Source3/RConn1
  Three-Phase Transformer (Two Windings)/RConn2 -- Controlled Voltage Source4/RConn1
  Three-Phase Transformer (Two Windings)/RConn3 -- Controlled Voltage Source5/RConn1

== system Assign_Task5and6/Task 5/VSC/VI measurement ==
  Current Measurement : spsCurrentMeasurementLib/Current Measurement  PhasorSimulation=off  OutputType=Complex  PSBequivalent=0
  Current Measurement1 : spsCurrentMeasurementLib/Current Measurement  PhasorSimulation=off  OutputType=Complex  PSBequivalent=0
  Current Measurement2 : spsCurrentMeasurementLib/Current Measurement  PhasorSimulation=off  OutputType=Complex  PSBequivalent=0
  Ground : spsGroundLib/Ground  LConnTagsString=a
  Ground1 : spsGroundLib/Ground  LConnTagsString=a
  Ground2 : spsGroundLib/Ground  LConnTagsString=a
  Mux : Mux  Inputs=3
  Mux1 : Mux  Inputs=3
  Voltage Measurement : spsVoltageMeasurementLib/Voltage Measurement  PhasorSimulation=off  OutputType=Complex  PSBequivalent=0
  Voltage Measurement1 : spsVoltageMeasurementLib/Voltage Measurement  PhasorSimulation=off  OutputType=Complex  PSBequivalent=0
  Voltage Measurement2 : spsVoltageMeasurementLib/Voltage Measurement  PhasorSimulation=off  OutputType=Complex  PSBequivalent=0
  A : PMIOPort  Side=Left
  B : PMIOPort  Port=2  Side=Left
  C : PMIOPort  Port=3  Side=Left
  a : PMIOPort  Port=4  Side=Right
  b : PMIOPort  Port=5  Side=Right
  c : PMIOPort  Port=6  Side=Right
  Vs : Outport
  Is : Outport  Port=2
  wires:
  Mux1/1 -> Is/1
  Mux/1 -> Vs/1
  Voltage Measurement1/1 -> Mux/2
  Voltage Measurement2/1 -> Mux/3
  Current Measurement2/1 -> Mux1/3
  Voltage Measurement/1 -> Mux/1
  Current Measurement/1 -> Mux1/1
  Current Measurement1/1 -> Mux1/2
  connections:
  Voltage Measurement/LConn1 -- Current Measurement/LConn1 -- A/RConn1
  Current Measurement2/LConn1 -- Voltage Measurement2/LConn1 -- C/RConn1
  Current Measurement1/LConn1 -- Voltage Measurement1/LConn1 -- B/RConn1
  Current Measurement1/RConn1 -- b/RConn1
  Current Measurement/RConn1 -- a/RConn1
  Ground/LConn1 -- Voltage Measurement/LConn2
  Current Measurement2/RConn1 -- c/RConn1
  Ground1/LConn1 -- Voltage Measurement1/LConn2
  Ground2/LConn1 -- Voltage Measurement2/LConn2

== system Assign_Task5and6/Task 5/VSC/VSC Control ==
  note: don't need to analyse this part
  note: don't need to analyse this part
  note: droop signal goes here
  Block : Inport
  Vabc : Inport  Port=2
  Iabc : Inport  Port=3
  Pset : Inport  Port=4
  Qset : Inport  Port=5
  "Control " : Subsystem  VariantControl=EMT_and_QEMT
  Measurement and PLL : Subsystem  VariantControl=EMT
  Modulation : Subsystem  VariantControl=EMT_AVG
  Mux : Mux  Inputs=2
  Ref : Outport
  m : Outport  Port=2
  wires:
  "Control "/1(vqd+-ref) -> Modulation/1(vqd+-*)
  [PQabc] -> Mux/2
  Modulation/1(Ref) -> Ref/1
  Vabc/1 -> Measurement and PLL/1(Vabc)
  Measurement and PLL/1(vqd+-) -> "Control "/3(vqd+-), [vqdpn]
  [theta] -> Modulation/2(theta)
  Iabc/1 -> Measurement and PLL/2(Iabc)
  Mux/1 -> m/1
  "Control "/2(m) -> Mux/1
  Pset/1 -> "Control "/1(Pset)
  Qset/1 -> "Control "/2(Qset)
  Block/1 -> "Control "/6(Block)
  Measurement and PLL/2(iqd+-) -> "Control "/4(iqd+-)
  Measurement and PLL/3(freq) -> "Control "/5(freq)
  Measurement and PLL/4(theta) -> [theta]
  Measurement and PLL/5(PQabc) -> [PQabc]

== system Assign_Task5and6/Task 5/VSC/output signals ==
  Vs : Inport
  Is : Inport  Port=2
  control : Inport  Port=3
  Bus Creator : BusCreator  Inputs=15
  Demux : Demux  Outputs=13
  m : Outport
  wires:
  Bus Creator/1 -> m/1
  control/1 -> Demux/1
  Vs/1 -> Bus Creator/1  "Vabc"
  Is/1 -> Bus Creator/2  "Iabc"
  Demux/1 -> Bus Creator/3  "vqp"
  Demux/2 -> Bus Creator/4  "vdp"
  Demux/3 -> Bus Creator/5  "vqn"
  Demux/4 -> Bus Creator/6  "vdn"
  Demux/5 -> Bus Creator/7  "iqp"
  Demux/6 -> Bus Creator/8  "idp"
  Demux/7 -> Bus Creator/9  "iqn"
  Demux/8 -> Bus Creator/10  "idn"
  Demux/9 -> Bus Creator/11  "f"
  Demux/10 -> Bus Creator/12  "Pdq"
  Demux/11 -> Bus Creator/13  "Qdq"
  Demux/12 -> Bus Creator/14  "Pabc"
  Demux/13 -> Bus Creator/15  "Qabc"

== system Assign_Task5and6/Task 6/Generator/Exciter ==
  note: The controller parameters provided by ENTSO-E
      | define different names for the parameters:
      |
      | ENTSO-E = IEEE Std 421.5-2005
      | Ta = Tc
      | Tb = Tb
      | K = Ka
      | Te = Ta
      | Emax = Vrmax
      | Emin = Vrmin
  note: The exciter model provided by ENTSO-E most similar to the IEEE is the Type AC4A excitation system model
  Vref : Inport
  Vt : Inport  Port=2
  Constant : Constant  Value=Vf0/K
  Saturation : Saturate  UpperLimit=Emax  LowerLimit=Emin
  Sum : Sum  Inputs=++-
  Transfer Fcn (with initial outputs) : simulink_extras/Additional Linear/Transfer Fcn (with initial outputs)  N=[K]  D=[Te 1]  Y0=Vf0  U0=Vf0/K
  Transfer Fcn (with initial outputs)1 : simulink_extras/Additional Linear/Transfer Fcn (with initial outputs)  N=[Ta 1]  D=[Tb 1]  Y0=Vf0/K  U0=Vf0/K
  Efd : Outport
  wires:
  Saturation/1 -> Efd/1
  Transfer Fcn (with initial outputs)1/1 -> Transfer Fcn (with initial outputs)/1
  Sum/1 -> Transfer Fcn (with initial outputs)1/1
  Transfer Fcn (with initial outputs)/1 -> Saturation/1
  Vt/1 -> Sum/3
  Vref/1 -> Sum/2
  Constant/1 -> Sum/1

== system Assign_Task5and6/Task 6/Generator/Turbine without governor ==
  note: mechanical power
  RefL : Inport
  Saturation : Saturate  UpperLimit=Vmax  LowerLimit=Vmin
  Saturation1 : Saturate  UpperLimit=1
  Transfer Fcn (with initial outputs)1 : simulink_extras/Additional Linear/Transfer Fcn (with initial outputs)  N=[T2 1]  D=[T3 1]  Y0=P0  U0=P0
  Transfer Fcn (with initial outputs)2 : simulink_extras/Additional Linear/Transfer Fcn (with initial outputs)  N=[1]  D=[T1 1]  Y0=P0  U0=P0
  Pm : Outport
  wires:
  Transfer Fcn (with initial outputs)1/1 -> Saturation1/1
  Saturation/1 -> Transfer Fcn (with initial outputs)1/1
  Transfer Fcn (with initial outputs)2/1 -> Saturation/1
  RefL/1 -> Transfer Fcn (with initial outputs)2/1
  Saturation1/1 -> Pm/1

== system Assign_Task5and6/Task 6/VSC/Electrical part ==
  Ref : Inport
  Controlled Voltage Source3 : spsControlledVoltageSourceLib/Controlled Voltage Source  Initialize=off  Source_Type=AC  Amplitude=Vhvpk  Phase=0  Frequency=fg  Measurements=None
  Controlled Voltage Source4 : spsControlledVoltageSourceLib/Controlled Voltage Source  Initialize=off  Source_Type=AC  Amplitude=Vhvpk  Phase=-2*pi/3  Frequency=fg  Measurements=None
  Controlled Voltage Source5 : spsControlledVoltageSourceLib/Controlled Voltage Source  Initialize=off  Source_Type=AC  Amplitude=Vhvpk  Phase=-4*pi/3  Frequency=fg  Measurements=None
  Demux1 : Demux  Outputs=3
  Ground : spsGroundLib/Ground  LConnTagsString=a
  Ground4 : spsGroundLib/Ground  LConnTagsString=a
  Ground5 : spsGroundLib/Ground  LConnTagsString=a
  Three-Phase Transformer (Two Windings) : spsThreePhaseTransformerTwoWindingsLib/Three-Phase Transformer (Two Windings)  Winding1Connection=Yg  Winding2Connection=Delta (D11)  CoreType=Three single-phase transformers  SetSaturation=off  Hysteresis=off  DataFile='hysteresis'  SetInitialFlux=off  Measurements=None  UNITS=pu  NominalPower=[Pconv , fg ]  Winding1=[Vhv, Rtpu/2, Xtpu/2]  Winding2=[Vmv, Rtpu/2, Xtpu/2]  Rm=5000  Lm=5000  L0=0.5  Saturation=[ 0,0 ; 0.0024,1.2 ; 1.0,1.52 ]  InitialFluxes=[ 0.8 , -0.8 , 0.7 ]  BreakLoop=off  DiscreteSolver=Trapezoidal iterative  DataType=off  TransfoNumber=1
  A : PMIOPort  Side=Left
  B : PMIOPort  Port=2  Side=Left
  C : PMIOPort  Port=3  Side=Left
  wires:
  Ref/1 -> Demux1/1
  Demux1/1 -> Controlled Voltage Source3/1
  Demux1/2 -> Controlled Voltage Source4/1
  Demux1/3 -> Controlled Voltage Source5/1
  connections:
  Ground/LConn1 -- Controlled Voltage Source3/LConn1
  Ground4/LConn1 -- Controlled Voltage Source4/LConn1
  Ground5/LConn1 -- Controlled Voltage Source5/LConn1
  Three-Phase Transformer (Two Windings)/LConn1 -- A/RConn1
  B/RConn1 -- Three-Phase Transformer (Two Windings)/LConn2
  Three-Phase Transformer (Two Windings)/LConn3 -- C/RConn1
  Three-Phase Transformer (Two Windings)/RConn1 -- Controlled Voltage Source3/RConn1
  Three-Phase Transformer (Two Windings)/RConn2 -- Controlled Voltage Source4/RConn1
  Three-Phase Transformer (Two Windings)/RConn3 -- Controlled Voltage Source5/RConn1

== system Assign_Task5and6/Task 6/VSC/VI measurement ==
  Current Measurement : spsCurrentMeasurementLib/Current Measurement  PhasorSimulation=off  OutputType=Complex  PSBequivalent=0
  Current Measurement1 : spsCurrentMeasurementLib/Current Measurement  PhasorSimulation=off  OutputType=Complex  PSBequivalent=0
  Current Measurement2 : spsCurrentMeasurementLib/Current Measurement  PhasorSimulation=off  OutputType=Complex  PSBequivalent=0
  Ground : spsGroundLib/Ground  LConnTagsString=a
  Ground1 : spsGroundLib/Ground  LConnTagsString=a
  Ground2 : spsGroundLib/Ground  LConnTagsString=a
  Mux : Mux  Inputs=3
  Mux1 : Mux  Inputs=3
  Voltage Measurement : spsVoltageMeasurementLib/Voltage Measurement  PhasorSimulation=off  OutputType=Complex  PSBequivalent=0
  Voltage Measurement1 : spsVoltageMeasurementLib/Voltage Measurement  PhasorSimulation=off  OutputType=Complex  PSBequivalent=0
  Voltage Measurement2 : spsVoltageMeasurementLib/Voltage Measurement  PhasorSimulation=off  OutputType=Complex  PSBequivalent=0
  A : PMIOPort  Side=Left
  B : PMIOPort  Port=2  Side=Left
  C : PMIOPort  Port=3  Side=Left
  a : PMIOPort  Port=4  Side=Right
  b : PMIOPort  Port=5  Side=Right
  c : PMIOPort  Port=6  Side=Right
  Vs : Outport
  Is : Outport  Port=2
  wires:
  Mux1/1 -> Is/1
  Mux/1 -> Vs/1
  Voltage Measurement1/1 -> Mux/2
  Voltage Measurement2/1 -> Mux/3
  Current Measurement2/1 -> Mux1/3
  Voltage Measurement/1 -> Mux/1
  Current Measurement/1 -> Mux1/1
  Current Measurement1/1 -> Mux1/2
  connections:
  Voltage Measurement/LConn1 -- Current Measurement/LConn1 -- A/RConn1
  Current Measurement2/LConn1 -- C/RConn1 -- Voltage Measurement2/LConn1
  Current Measurement1/LConn1 -- Voltage Measurement1/LConn1 -- B/RConn1
  Current Measurement1/RConn1 -- b/RConn1
  Current Measurement/RConn1 -- a/RConn1
  Ground/LConn1 -- Voltage Measurement/LConn2
  Current Measurement2/RConn1 -- c/RConn1
  Ground1/LConn1 -- Voltage Measurement1/LConn2
  Ground2/LConn1 -- Voltage Measurement2/LConn2

== system Assign_Task5and6/Task 6/VSC/VSC Control ==
  note: don't need to analyse this part
  note: don't need to analyse this part
  note: droop signal goes here
  Block : Inport
  Vabc : Inport  Port=2
  Iabc : Inport  Port=3
  Pset : Inport  Port=4
  Qset : Inport  Port=5
  "Control " : Subsystem  VariantControl=EMT_and_QEMT
  Measurement and PLL : Subsystem  VariantControl=EMT
  Modulation : Subsystem  VariantControl=EMT_AVG
  Mux : Mux  Inputs=2
  Ref : Outport
  m : Outport  Port=2
  wires:
  "Control "/1(vqd+-ref) -> Modulation/1(vqd+-*)
  [PQabc] -> Mux/2
  Modulation/1(Ref) -> Ref/1
  Vabc/1 -> Measurement and PLL/1(Vabc)
  Measurement and PLL/1(vqd+-) -> "Control "/3(vqd+-), [vqdpn]
  [theta] -> Modulation/2(theta)
  Iabc/1 -> Measurement and PLL/2(Iabc)
  Mux/1 -> m/1
  "Control "/2(m) -> Mux/1
  Pset/1 -> "Control "/1(Pset)
  Qset/1 -> "Control "/2(Qset)
  Block/1 -> "Control "/6(Block)
  Measurement and PLL/2(iqd+-) -> "Control "/4(iqd+-)
  Measurement and PLL/3(freq) -> "Control "/5(freq)
  Measurement and PLL/4(theta) -> [theta]
  Measurement and PLL/5(PQabc) -> [PQabc]

== system Assign_Task5and6/Task 6/VSC/output signals ==
  Vs : Inport
  Is : Inport  Port=2
  control : Inport  Port=3
  Bus Creator : BusCreator  Inputs=15
  Demux : Demux  Outputs=13
  m : Outport
  wires:
  Bus Creator/1 -> m/1
  control/1 -> Demux/1
  Vs/1 -> Bus Creator/1  "Vabc"
  Is/1 -> Bus Creator/2  "Iabc"
  Demux/1 -> Bus Creator/3  "vqp"
  Demux/2 -> Bus Creator/4  "vdp"
  Demux/3 -> Bus Creator/5  "vqn"
  Demux/4 -> Bus Creator/6  "vdn"
  Demux/5 -> Bus Creator/7  "iqp"
  Demux/6 -> Bus Creator/8  "idp"
  Demux/7 -> Bus Creator/9  "iqn"
  Demux/8 -> Bus Creator/10  "idn"
  Demux/9 -> Bus Creator/11  "f"
  Demux/10 -> Bus Creator/12  "Pdq"
  Demux/11 -> Bus Creator/13  "Qdq"
  Demux/12 -> Bus Creator/14  "Pabc"
  Demux/13 -> Bus Creator/15  "Qabc"
